simulink model "bang_bang_hist_DI_PD"  (R2016a)
settings: Solver=ode45  StartTime=0.0  StopTime=10  MaxStep=1e-5  RelTol=1e-3
values from neighbouring files (symbols this model uses):
  a = - C.Z{1}    [actividad3.m]
  K = 5    [actividad3.m]    (also in actividad3PID.m)
  Kc = C.K    [actividad3.m]
  lineal = 0    [actividad3.m]
  M = Kc    [actividad3.m]
  p1 = 3    [actividad3.m]    (also in actividad3PID.m)
  p2 = -1    [actividad3.m]    (also in actividad3PID.m)
  T = (Kc*K)/100    [actividad3.m]    (also in actividad3PID.m = 1)
settings Model: Creator=Usuario  LastModifiedBy=PC
settings DataIOCC: SaveFormat=Array  SignalLoggingSaveFormat=ModelDataLogs
settings OptimizationCC: BlockReduction=off  BooleanDataType=off  InitFltsAndDblsToZero=on
settings DebuggingCC: SaveWithParameterizedLinksMsg=none  UnderspecifiedInitializationDetection=Classic  MergeDetectMultiDrivingBlocksExec=none  SignalResolutionControl=TryResolveAllWithWarning  MultiTaskDSMMsg=warning  MultiTaskCondExecSysMsg=none  FcnCallInpInsideContextMsg=UseLocalSettings
settings HardwareCC: ProdBitPerPointer=32  ProdLargestAtomicFloat=None  ProdIntDivRoundTo=Undefined  ProdEndianess=Unspecified  ProdWordSize=32  ProdHWDeviceType=32-bit Generic  TargetUnknown=on
settings ModelReferenceCC: PropagateSignalLabelsOutOfModel=off
settings RTWCC: Description=Generic Real-Time Target
settings GRTTargetCC: TargetFcnLib=ansi_tfl_tmw.mat  CombineOutputUpdateFcns=off  GRTInterface=on
settings ConfigComp: CovModelRefEnable=Off  CovSFcnEnable=off

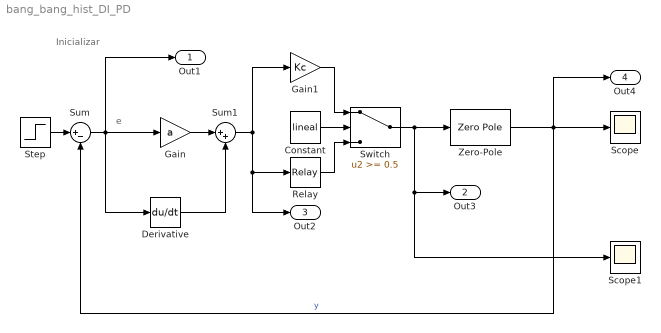
== system bang_bang_hist_DI_PD ==
  note: Inicializar
  note: e
  Constant : Constant  Value=lineal
  Derivative : Derivative
  Gain : Gain  Gain=a
  Gain1 : Gain  Gain=Kc
  Relay : Relay  OnSwitchValue=T  OffSwitchValue=-T  OnOutputValue=M  OffOutputValue=-M
  Scope : Scope
  Scope1 : Scope
  Step : Step  Time=0  SampleTime=0
  Sum : Sum  Inputs=|+-  SaturateOnIntegerOverflow=on  InputSameDT=on  OutDataTypeStr=Inherit: Same as first input
  Sum1 : Sum  Inputs=|++
  Switch : Switch  Threshold=0.5
  Zero-Pole : ZeroPole  Zeros=[]  Poles=[p2 p1]  Gain=[K]
  Out1 : Outport
  Out3 : Outport  Port=2
  Out2 : Outport  Port=3
  Out4 : Outport  Port=4
  wires:
  Zero-Pole/1 -> Out4/1, Sum/2, Scope/1  "y"
  Step/1 -> Sum/1
  Derivative/1 -> Sum1/2
  Sum/1 -> Gain/1, Out1/1, Derivative/1
  Gain/1 -> Sum1/1
  Relay/1 -> Switch/3
  Switch/1 -> Out3/1, Scope1/1, Zero-Pole/1
  Sum1/1 -> Out2/1, Relay/1, Gain1/1
  Gain1/1 -> Switch/1
  Constant/1 -> Switch/2
